simulink model "observador_reducido"  (R2020a)
settings: Solver=VariableStepAuto  StartTime=0.0  StopTime=10.0  RelTol=1e-3
undefined symbols (not defined in the file): Jl, Jm, Ke_theta, Ke_w, r
settings Model: Creator=Ferran  LastModifiedBy=Ferran

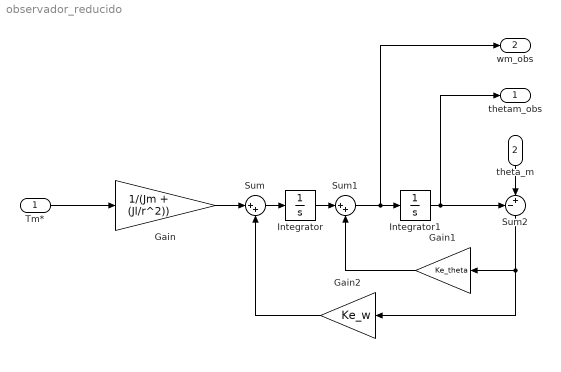
== system observador_reducido ==
  Tm* : Inport
  theta_m : Inport  Port=2
  Gain : Gain  Gain=1/(Jm + (Jl/r^2))
  Gain1 : Gain  Gain=Ke_theta
  Gain2 : Gain  Gain=Ke_w
  Integrator : Integrator
  Integrator1 : Integrator
  Sum : Sum  Inputs=|++
  Sum1 : Sum  Inputs=|++
  Sum2 : Sum  Inputs=-+|
  thetam_obs : Outport
  wm_obs : Outport  Port=2
  wires:
  Tm*/1 -> Gain/1
  Gain/1 -> Sum/1
  Sum/1 -> Integrator/1
  Integrator/1 -> Sum1/1
  Sum1/1 -> wm_obs/1, Integrator1/1
  theta_m/1 -> Sum2/2
  Sum2/1 -> Gain2/1, Gain1/1
  Gain1/1 -> Sum1/2
  Gain2/1 -> Sum/2
  Integrator1/1 -> thetam_obs/1, Sum2/1
